simulink model "untitled"  (R2017a)
settings: Solver=ode8  StartTime=0.0  StopTime=3  FixedStep=1e-5  RelTol=1e-3  EnableMultiTasking=on
settings Model: Creator=Administrator  LastModifiedBy=Administrator
settings DataIOCC: LimitDataPoints=on  SaveFormat=Array
settings OptimizationCC: LifeSpan=inf
settings DebuggingCC: SolverPrmCheckMsg=warning  MultiTaskDSMMsg=warning  MultiTaskCondExecSysMsg=none  FcnCallInpInsideContextMsg=warning  SFUnexpectedBacktrackingDiag=warning  SFNoUnconditionalDefaultTransitionDiag=warning  SFExecutionAtInitializationDiag=none
settings HardwareCC: ProdBitPerPointer=32  ProdBitPerSizeT=32  ProdBitPerPtrDiffT=32  ProdLargestAtomicFloat=None  ProdIntDivRoundTo=Undefined  ProdEndianess=Unspecified  ProdWordSize=32  ProdHWDeviceType=32-bit Generic
settings ModelReferenceCC: PropagateSignalLabelsOutOfModel=off
settings GRTTargetCC: TargetLangStandard=C89/C90 (ANSI)  GeneratePreprocessorConditionals=Disable all
settings ConfigComp: CovMetricSettings=dw  CovHtmlReporting=on  CovSaveCumulativeToWorkspaceVar=on  CovSaveSingleToWorkspaceVar=on  CovExternalEMLEnable=off

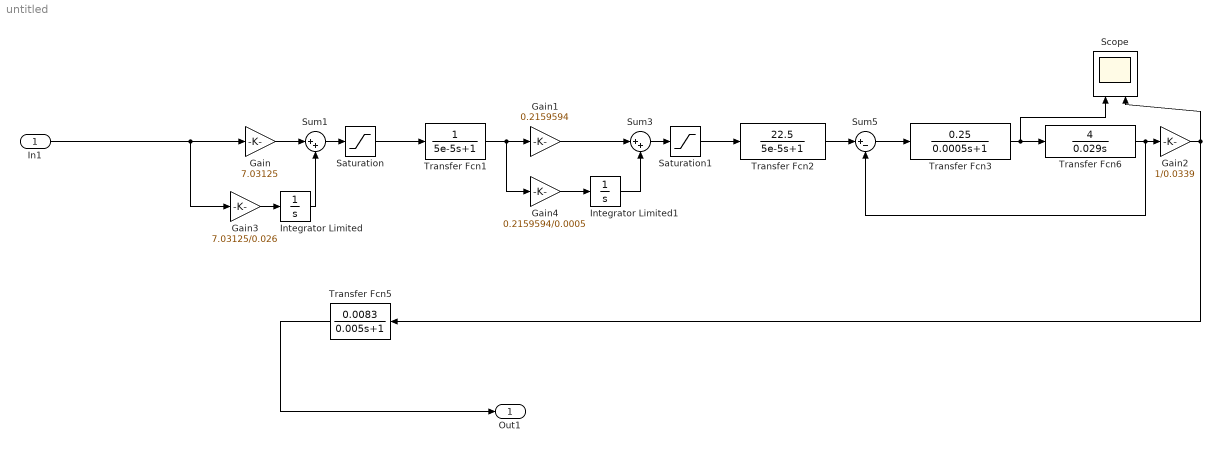
== system untitled ==
  In1 : Inport
  Gain : Gain  Gain=7.03125
  Gain1 : Gain  Gain=0.2159594
  Gain2 : Gain  Gain=1/0.0339
  Gain3 : Gain  Gain=7.03125/0.026
  Gain4 : Gain  Gain=0.2159594/0.0005
  Integrator Limited : Integrator  LimitOutput=on  UpperSaturationLimit=10  LowerSaturationLimit=-10
  Integrator Limited1 : Integrator  LimitOutput=on  UpperSaturationLimit=15  LowerSaturationLimit=-15
  Saturation : Saturate  UpperLimit=10  LowerLimit=-10
  Saturation1 : Saturate  UpperLimit=15  LowerLimit=-15
  Scope : Scope  NumInputPorts=2
  Sum1 : Sum  Inputs=|++
  Sum3 : Sum  Inputs=|++
  Sum5 : Sum  Inputs=|+-
  Transfer Fcn1 : TransferFcn  Denominator=[5e-5 1]
  Transfer Fcn2 : TransferFcn  Numerator=[22.5]  Denominator=[5e-5 1]
  Transfer Fcn3 : TransferFcn  Numerator=[0.25]  Denominator=[0.0005 1]
  Transfer Fcn5 : TransferFcn  Numerator=[0.0083]  Denominator=[0.005 1]
  Transfer Fcn6 : TransferFcn  Numerator=[4]  Denominator=[0.029 0]
  Out1 : Outport
  wires:
  Sum1/1 -> Saturation/1
  Saturation/1 -> Transfer Fcn1/1
  Transfer Fcn1/1 -> Gain1/1, Gain4/1
  Gain1/1 -> Sum3/1
  Gain/1 -> Sum1/1
  Gain3/1 -> Integrator Limited/1
  Integrator Limited/1 -> Sum1/2
  Gain4/1 -> Integrator Limited1/1
  Integrator Limited1/1 -> Sum3/2
  Sum3/1 -> Saturation1/1
  Saturation1/1 -> Transfer Fcn2/1
  Transfer Fcn2/1 -> Sum5/1
  Sum5/1 -> Transfer Fcn3/1
  Transfer Fcn3/1 -> Scope/1, Transfer Fcn6/1
  Gain2/1 -> Scope/2, Transfer Fcn5/1
  Transfer Fcn6/1 -> Sum5/2, Gain2/1
  In1/1 -> Gain/1, Gain3/1
  Transfer Fcn5/1 -> Out1/1
